simulink model "sistema_controlador_digital"  (R2018a)
settings: Solver=VariableStepAuto  StartTime=0.0  StopTime=10.0  RelTol=1e-3
values from neighbouring files (symbols this model uses):
  Kd = .5    (= 0.5)    [teste_bw.m]    (also in teste_feedback.m = 1; teste_sinal_de_controle.m = coef(3); teste_tf.m)
  Ki = 0.3    [teste_bw.m]    (also in teste_feedback.m = 1; teste_sinal_de_controle.m = coef(2); teste_tf.m)
  Kp = 1    [parametros_pid.m]    (also in teste_bw.m = 3; teste_feedback.m; teste_sinal_de_controle.m = coef(1); teste_tf.m = 3)
  wn = 8.036118730219977    (= 8.03611873022)    [entrada_arbitraria.m]    (also in entrada_arbitrária.m; parametros_pid.m; teste_aleatorio_input.m; teste_bw.m = 1)
  zeta = 0.900733958553509    (= 0.900733958554)    [entrada_arbitraria.m]    (also in entrada_arbitrária.m; parametros_pid.m; teste_aleatorio_input.m; teste_bw.m = 1)
libraries: simulink x1
settings Model: Creator=Eric Moretti  LastModifiedBy=Eric Moretti

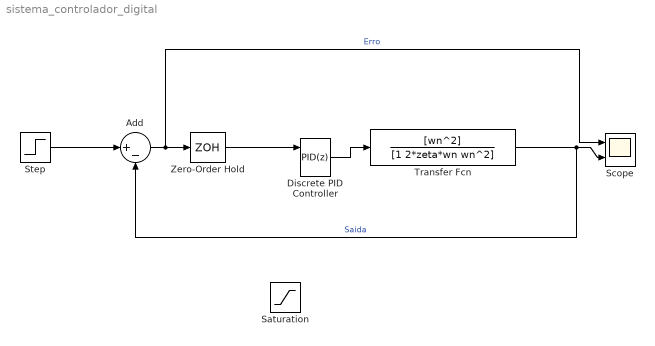
== system sistema_controlador_digital ==
  Add : Sum  Inputs=|+-
  Discrete PID Controller : simulink/Continuous/PID Controller  Controller=PID  TimeDomain=Discrete-time  SampleTime=0.1  IntegratorMethod=Forward Euler  FilterMethod=Forward Euler  Form=Parallel  UseFilter=off  ControllerParametersSource=internal  P=Kp  I=Ki  D=Kd  N=100  InitialConditionSource=external  InitialConditionForIntegrator=0  InitialConditionForFilter=0  ExternalReset=none  LimitOutput=off  UpperSaturationLimit=inf  LowerSaturationLimit=-inf  LinearizeAsGain=off  AntiWindupMode=none  Kb=1  TrackingMode=off  Kt=1  PParamMin=[]  PParamMax=[]  IParamMin=[]  IParamMax=[]  DParamMin=[]  DParamMax=[]  NParamMin=[]  NParamMax=[]  KbParamMin=[]  KbParamMax=[]  KtParamMin=[]  KtParamMax=[]  POutMin=[]  POutMax=[]  IOutMin=[]  IOutMax=[]  DOutMin=[]  DOutMax=[]  NOutMin=[]  NOutMax=[]  KbOutMin=[]  KbOutMax=[]  KtOutMin=[]  KtOutMax=[]  IntegratorOutMin=[]  IntegratorOutMax=[]  FilterOutMin=[]  FilterOutMax=[]  SumOutMin=[]  SumOutMax=[]  SumI1OutMin=[]  SumI1OutMax=[]  SumI2OutMin=[]  SumI2OutMax=[]  SumI3OutMin=[]  SumI3OutMax=[]  SumDOutMin=[]  SumDOutMax=[]  SaturationOutMin=[]  SaturationOutMax=[]  IntegratorContinuousStateAttributes=''  IntegratorStateMustResolveToSignalObject=off  IntegratorRTWStateStorageClass=Auto  FilterContinuousStateAttributes=''  FilterStateMustResolveToSignalObject=off  FilterRTWStateStorageClass=Auto  DifferentiatorICPrevScaledInput=0  DifferentiatorOutMin=[]  DifferentiatorOutMax=[]  FilterDiffOutCoefMin=[]  FilterDiffOutCoefMax=[]  SumDenOutMin=[]  SumDenOutMax=[]  SumNumOutMin=[]  SumNumOutMax=[]  ReciprocalOutMin=[]  ReciprocalOutMax=[]  DivideOutMin=[]  DivideOutMax=[]  TunerSelectOption=Transfer Function Based (PID Tuner App)
  Saturation : Saturate  UpperLimit=1  LowerLimit=0
  Scope : Scope  NumInputPorts=2
  Step : Step  Time=0  SampleTime=0
  Transfer Fcn : TransferFcn  Numerator=[wn^2]  Denominator=[1 2*zeta*wn wn^2]
  Zero-Order Hold : ZeroOrderHold  SampleTime=0.1
  wires:
  Transfer Fcn/1 -> Add/2, Scope/2  "Saida"
  Add/1 -> Zero-Order Hold/1, Scope/1  "Erro"
  Zero-Order Hold/1 -> Discrete PID Controller/1
  Discrete PID Controller/1 -> Transfer Fcn/1
  Step/1 -> Add/1
